simulink model "Thruster_Characteristics"  (R2023b)
settings: Solver=VariableStepAuto  StartTime=0.0  StopTime=10  RelTol=1e-3
settings Model: Creator=Ottol  LastModifiedBy=Ottol
settings ModelReferenceCC: EnableRefExpFcnMdlSchedulingChecks=on

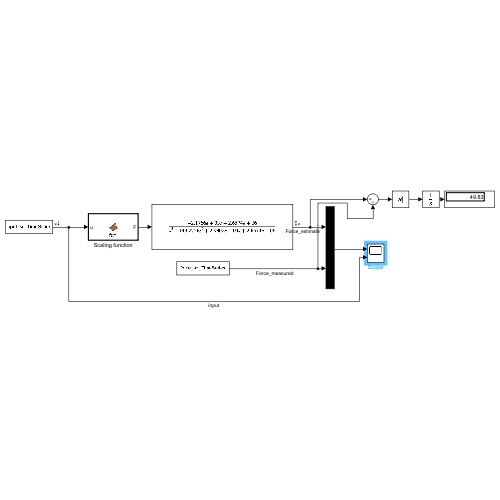
[thumbnail: Simulink's stored preview of the top-level diagram]
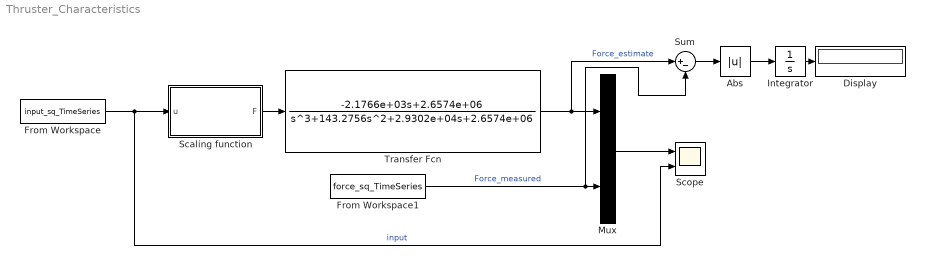
== system Thruster_Characteristics ==
  Abs : Abs  SaturateOnIntegerOverflow=off
  Display : Display
  From Workspace : FromWorkspace  VariableName=input_sq_TimeSeries  SampleTime=0.002
  From Workspace1 : FromWorkspace  VariableName=force_sq_TimeSeries  SampleTime=0.002
  Integrator : Integrator
  Mux : Mux  Inputs=2
  Scaling function : MATLAB Function  TreatAsAtomicUnit=on
  Scope : Scope  NumInputPorts=2
  Sum : Sum  Inputs=|+-
  Transfer Fcn : TransferFcn  Numerator=[0 0 -2.1766e+03 2.6574e+06]  Denominator=[1 143.2756 2.9302e+04 2.6574e+06]
  wires:
  Scaling function/1(F) -> Transfer Fcn/1
  Transfer Fcn/1 -> Sum/1, Mux/1  "Force_estimate"
  Mux/1 -> Scope/1
  From Workspace/1 -> Scope/2, Scaling function/1(u)  "input"
  From Workspace1/1 -> Sum/2, Mux/2  "Force_measured"
  Sum/1 -> Abs/1
  Abs/1 -> Integrator/1
  Integrator/1 -> Display/1

== matlab function Thruster_Characteristics/Scaling function ==
  data: u input; F output
function F = fcn(u)
%16V
%p =  [-148.575215521583	-6.01951344606880	347.062027953365	14.7939725163702	-299.865931981745	-13.0166356354772	134.177990099770	10.1629233711657	12.7092879704266	-0.0232735493306251];

%14 V
p = [-111.940783464042	-6.65861599537878	269.823430407384	13.8659958797022	-243.064927768226	-10.2880091499065	114.063389337106	8.09188399656116	10.6145211900378	-0.00];

F = polyval(p,u);
